simulink model "P6_Modelo_4_15_MotorCompleto"  (R2021b)
settings: Solver=FixedStepAuto  StartTime=0.0  StopTime=15  FixedStep=1e-4  RelTol=1e-3  EnableMultiTasking=on
undefined symbols (not defined in the file): C, f, F, G, K, Ki, L, T, thetaref
libraries: mbedblockslib x6, simulink x2
settings Model: ExtModeTrigDuration=10  Creator=Usuario  LastModifiedBy=abierto
settings OptimizationCC: EnhancedBackFolding=on  PassReuseOutputArgsAs=Individual arguments  ZeroExternalMemoryAtStartup=off  ZeroInternalMemoryAtStartup=off  MaxStackSize=64  OptimizeBlockOrder=speed  DifferentSizesBufferReuse=on  OptimizationCustomize=off  EfficientTunableParamExpr=on
settings DebuggingCC: ParameterTunabilityLossMsg=error  UnconnectedInputMsg=none  UnconnectedOutputMsg=none  UnconnectedLineMsg=none
settings HardwareCC: ProdBitPerPointer=32  ProdBitPerSizeT=32  ProdBitPerPtrDiffT=32  ProdLargestAtomicInteger=Long  ProdLargestAtomicFloat=Double  ProdWordSize=32  ProdLongLongMode=on  ProdHWDeviceType=ARM Compatible->ARM Cortex
settings ModelReferenceCC: EnableRefExpFcnMdlSchedulingChecks=off
settings SFSimCC: MATLABDynamicMemAlloc=off
settings RTWCC: Description=Embedded Coder  SystemTargetFile=ert.tlc  HardwareBoard=STM32 Nucleo F411RE  TemplateMakefile=ert_default_tmf  Toolchain=GNU Tools for ARM Embedded Processors  DLArmComputeVersion=20.02.1
settings CodeAppCC: ForceParamTrailComments=on  IgnoreCustomStorageClasses=off  OperatorAnnotations=on  SimulinkDataObjDesc=on  SFDataObjDesc=on  InsertBlockDesc=on
settings ERTTargetCC: SupportContinuousTime=on  ExtModeTransport=3  ExtModeStaticAlloc=on  ExtModeStaticAllocSize=2000  ExtModeMexFile=ext_xcp  ExtModeIntrfLevel=Level2 - Open

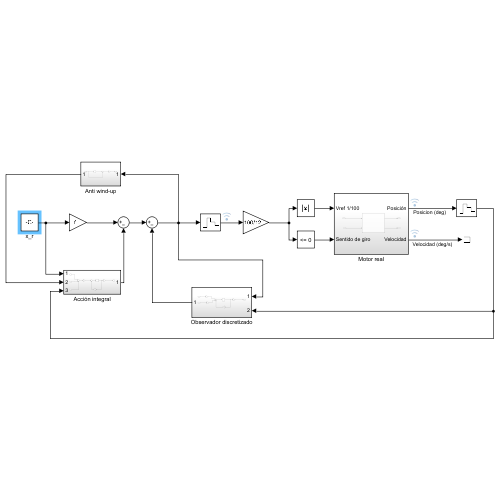
[thumbnail: Simulink's stored preview of the top-level diagram]
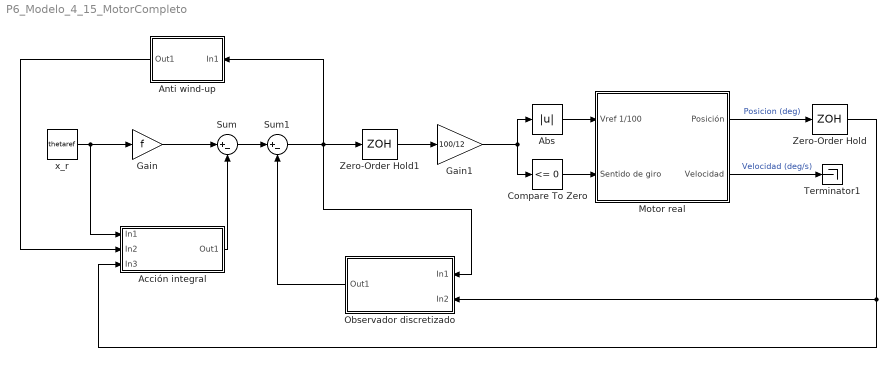
== system P6_Modelo_4_15_MotorCompleto ==
  Abs : Abs
  Acción integral : Subsystem
  Anti wind-up : Subsystem
      settings: PortSchema="{\"entries\":[{\"content\":{\"sides\":[{\"content\":{\"connectorIds\":[\"Out1\"]},\"type\":\"ConnectorPlacement.EquallySpacedRectSide\",\"uuid\":\"749271f6-54f1-4f24-9600-ea499e928faa\"},{\"content\":{\"connectorIds\":[\"In1\"],\"side\":\"RIGHT\"},\"type\":\"ConnectorPlacement.EquallySpacedRectSide\",\"uuid\":\"ee9435a8-dbe1-40c1-a065-bb113cdbdbca\"},{\"content\":{\"side\":\"TOP\"},\"type\":\"ConnectorPlacement.EquallySpacedRectSide\",\"uuid\":\"52b3e7c6-e784-4572-ae84-cac30e4683ac\"},{\"content\":{\"side\":\"BOTTOM\"},\"type\":\"ConnectorPlacement.EquallySpacedRectSide\",\"uuid\":\"d0a8c3d0-652d-41d0-89a7-692f2407b8d7\"}]},\"type\":\"ConnectorPlacement.EquallySpacedConnector\",\"uuid\":\"8824af27-d422-4acb-9a8e-58c102130d82\"}],\"packageUris\":[\"http://schema.mathworks.com/mf0/Connector/R2020b\"],\"version\":\"1.0\"}"
  Compare To Zero : simulink/Logic and Bit Operations/Compare To Zero  relop=<=  OutDataTypeStr=boolean
  Gain : Gain  Gain=f
  Gain1 : Gain  Gain=100/12
  Motor real : Subsystem
  Observador discretizado : Subsystem
      settings: PortSchema="{\"entries\":[{\"content\":{\"sides\":[{\"content\":{\"connectorIds\":[\"Out1\"]},\"type\":\"ConnectorPlacement.EquallySpacedRectSide\",\"uuid\":\"6435dc11-cf89-4f05-818f-b2f26a414da8\"},{\"content\":{\"connectorIds\":[\"In1\",\"In2\"],\"side\":\"RIGHT\"},\"type\":\"ConnectorPlacement.EquallySpacedRectSide\",\"uuid\":\"1bf393f3-1ca4-48a3-bb68-aa08f87c5096\"},{\"content\":{\"side\":\"TOP\"},\"type\":\"ConnectorPlacement.EquallySpacedRectSide\",\"uuid\":\"50c53087-a72d-4dad-8f1b-14b045676baf\"}]},\"type\":\"ConnectorPlacement.EquallySpacedConnector\",\"uuid\":\"309140f8-57ab-4a40-a8b6-79c71290e69d\"}],\"packageUris\":[\"http://schema.mathworks.com/mf0/Connector/R2020b\"],\"version\":\"1.0\"}"
  Sum : Sum  Inputs=|+-
  Sum1 : Sum  Inputs=|+-
  Terminator1 : Terminator
  Zero-Order Hold : ZeroOrderHold  SampleTime=0.0001
  Zero-Order Hold1 : ZeroOrderHold  SampleTime=0.0001
  x_r : Constant  Value=thetaref
  wires:
  Motor real/1(Posición) -> Zero-Order Hold/1  "Posicion (deg)"
  Motor real/2(Velocidad) -> Terminator1/1  "Velocidad (deg/s)"
  Sum/1 -> Sum1/1
  Abs/1 -> Motor real/1(Vref 1/100)
  Compare To Zero/1 -> Motor real/2(Sentido de giro)
  Zero-Order Hold1/1 -> Gain1/1
  Sum1/1 -> Anti wind-up/1(In1), Observador discretizado/1(In1), Zero-Order Hold1/1
  x_r/1 -> Acción integral/1(In1), Gain/1
  Gain/1 -> Sum/1
  Zero-Order Hold/1 -> Acción integral/3(In3), Observador discretizado/2(In2)
  Observador discretizado/1(Out1) -> Sum1/2
  Acción integral/1(Out1) -> Sum/2
  Anti wind-up/1(Out1) -> Acción integral/2(In2)
  Gain1/1 -> Abs/1, Compare To Zero/1

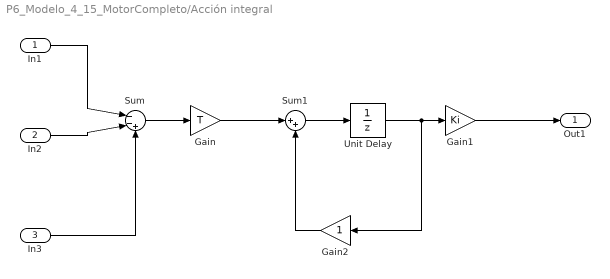
== system P6_Modelo_4_15_MotorCompleto/Acción integral ==
  In1 : Inport
  In2 : Inport  Port=2
  In3 : Inport  Port=3
  Gain : Gain  Gain=T
  Gain1 : Gain  Gain=Ki
  Gain2 : Gain
  Sum : Sum  Inputs=|--+
  Sum1 : Sum  Inputs=|++
  Unit Delay : UnitDelay  SampleTime=0.0001  HasFrameUpgradeWarning=on
  Out1 : Outport
  wires:
  In1/1 -> Sum/1
  In2/1 -> Sum/2
  In3/1 -> Sum/3
  Sum/1 -> Gain/1
  Gain/1 -> Sum1/1
  Sum1/1 -> Unit Delay/1
  Unit Delay/1 -> Gain2/1, Gain1/1
  Gain1/1 -> Out1/1
  Gain2/1 -> Sum1/2

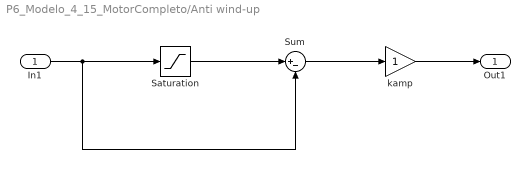
== system P6_Modelo_4_15_MotorCompleto/Anti wind-up ==
  In1 : Inport
  Saturation : Saturate
  Sum : Sum  Inputs=|+-
  kamp : Gain
  Out1 : Outport
  wires:
  In1/1 -> Sum/2, Saturation/1
  Saturation/1 -> Sum/1
  Sum/1 -> kamp/1
  kamp/1 -> Out1/1

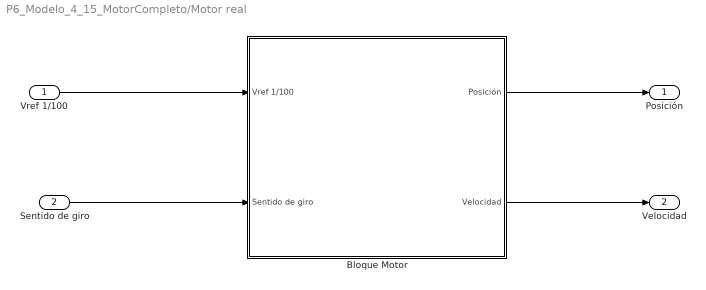
== system P6_Modelo_4_15_MotorCompleto/Motor real ==
  Vref 1/100 : Inport
  Sentido de giro : Inport  Port=2
  Bloque Motor : Subsystem
  Posición : Outport
  Velocidad : Outport  Port=2
  wires:
  Bloque Motor/1(Posición) -> Posición/1
  Bloque Motor/2(Velocidad) -> Velocidad/1
  Vref 1/100/1 -> Bloque Motor/1(Vref 1/100)
  Sentido de giro/1 -> Bloque Motor/2(Sentido de giro)

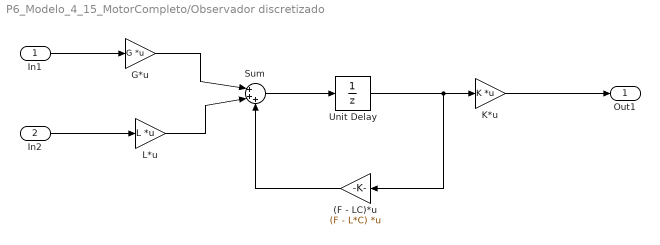
== system P6_Modelo_4_15_MotorCompleto/Observador discretizado ==
  In1 : Inport
  In2 : Inport  Port=2
  (F - LC)*u : Gain  Gain=(F - L*C)  Multiplication=Matrix(K*u)
  G*u : Gain  Gain=G  Multiplication=Matrix(K*u)
  K*u : Gain  Gain=K  Multiplication=Matrix(K*u)
  L*u : Gain  Gain=L  Multiplication=Matrix(K*u)
  Sum : Sum  Inputs=|+++
  Unit Delay : UnitDelay  SampleTime=0.0001  HasFrameUpgradeWarning=on
  Out1 : Outport
  wires:
  In1/1 -> G*u/1
  In2/1 -> L*u/1
  G*u/1 -> Sum/1
  L*u/1 -> Sum/2
  Sum/1 -> Unit Delay/1
  Unit Delay/1 -> (F - LC)*u/1, K*u/1
  K*u/1 -> Out1/1
  (F - LC)*u/1 -> Sum/3

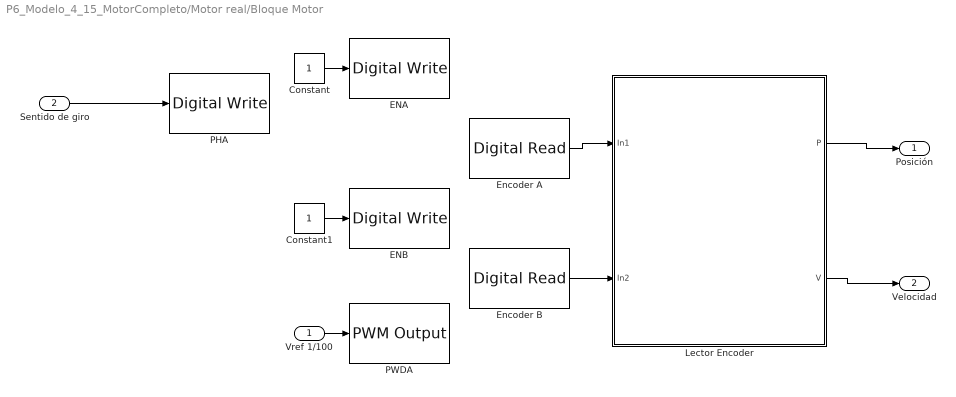
== system P6_Modelo_4_15_MotorCompleto/Motor real/Bloque Motor ==
  Vref 1/100 : Inport
  Sentido de giro : Inport  Port=2
  Constant : Constant
  Constant1 : Constant
  ENA : mbedblockslib/Digital Write  Pin=D2  Direction=output
      settings: SourceProductBaseCode=MICROBIT,NUCLEO,STMICRODIS
  ENB : mbedblockslib/Digital Write  Pin=D11  Direction=output
      settings: SourceProductBaseCode=MICROBIT,NUCLEO,STMICRODIS
  Encoder A : mbedblockslib/Digital Read  Pin=A1  Direction=input  SampleTime=0.0001
      settings: SourceProductBaseCode=MICROBIT,NUCLEO,STMICRODIS
  Encoder B : mbedblockslib/Digital Read  Pin=A0  Direction=input  SampleTime=0.0001
      settings: SourceProductBaseCode=MICROBIT,NUCLEO,STMICRODIS
  Lector Encoder : Subsystem
  PHA : mbedblockslib/Digital Write  Pin=D3  Direction=output
      settings: SourceProductBaseCode=MICROBIT,NUCLEO,STMICRODIS
  PWDA : mbedblockslib/PWM Output  Pin=D5  EnableInputFrequency=off  InitialFrequency=5000  InitialDutyCycle=50  NotificationType=None
      settings: SourceProductBaseCode=MICROBIT,NUCLEO,STMICRODIS
  Posición : Outport
  Velocidad : Outport  Port=2
  wires:
  Sentido de giro/1 -> PHA/1
  Constant/1 -> ENA/1
  Constant1/1 -> ENB/1
  Vref 1/100/1 -> PWDA/1
  Encoder A/1 -> Lector Encoder/1(In1)
  Encoder B/1 -> Lector Encoder/2(In2)
  Lector Encoder/1(P) -> Posición/1
  Lector Encoder/2(V) -> Velocidad/1

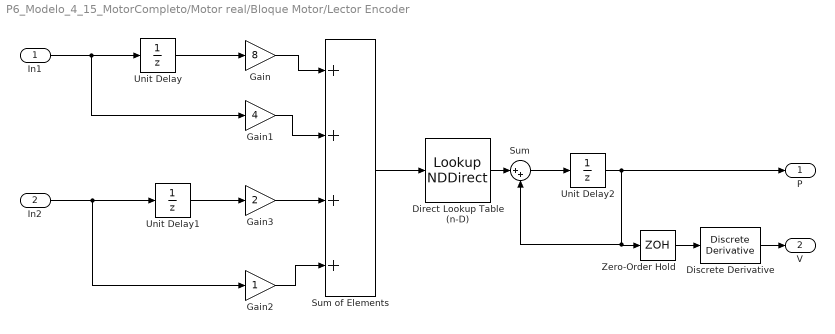
== system P6_Modelo_4_15_MotorCompleto/Motor real/Bloque Motor/Lector Encoder ==
  In1 : Inport
  In2 : Inport  Port=2
  Direct Lookup Table (n-D) : LookupNDDirect  NumberOfTableDimensions=1  Table=[0,-1,1,0,1,0,0,-1,-1,0,0,1,0,1,-1,0]
  Discrete Derivative : simulink/Discrete/Discrete Derivative  gainval=1.0  ICPrevScaledInput=0.0  OutMin=[]  OutMax=[]  OutDataType=fixdt(1, 16)  OutScaling=2^-10  DoSatur=off
  Gain : Gain  Gain=8
  Gain1 : Gain  Gain=4
  Gain2 : Gain
  Gain3 : Gain  Gain=2
  Sum : Sum  Inputs=|++
  Sum of Elements : Sum  Inputs=++++  OutDataTypeStr=double
  Unit Delay : UnitDelay  SampleTime=-1  HasFrameUpgradeWarning=on
  Unit Delay1 : UnitDelay  SampleTime=-1  HasFrameUpgradeWarning=on
  Unit Delay2 : UnitDelay  SampleTime=-1  HasFrameUpgradeWarning=on
  Zero-Order Hold : ZeroOrderHold  SampleTime=0.01
  P : Outport
  V : Outport  Port=2
  wires:
  In1/1 -> Gain1/1, Unit Delay/1
  In2/1 -> Gain2/1, Unit Delay1/1
  Unit Delay/1 -> Gain/1
  Unit Delay1/1 -> Gain3/1
  Gain/1 -> Sum of Elements/1
  Gain1/1 -> Sum of Elements/2
  Gain3/1 -> Sum of Elements/3
  Gain2/1 -> Sum of Elements/4
  Sum of Elements/1 -> Direct Lookup Table (n-D)/1
  Direct Lookup Table (n-D)/1 -> Sum/1
  Sum/1 -> Unit Delay2/1
  Unit Delay2/1 -> Sum/2, Zero-Order Hold/1, P/1
  Discrete Derivative/1 -> V/1
  Zero-Order Hold/1 -> Discrete Derivative/1
